simulink model "TP7_EJ3_espacio_estados"  (R2020a)
settings: Solver=VariableStepAuto  StartTime=0.0  StopTime=60  MaxStep=0.01  RelTol=1e-3
values from neighbouring files (symbols this model uses):
  A = [0 1 0 0 ... (first row only)    [TP7_EJ3_matrices.m]    (also in TP7_EJ6_matrices.m; TP7_EJ8.m)
  B = [0 0 0 1/m2]'    [TP7_EJ3_matrices.m]    (also in TP7_EJ6_matrices.m; TP7_EJ8.m = [0 0 0 k2/m2]')
  C1 = [1 0 0 0]    [TP7_EJ3_matrices.m]
  C2 = [0 0 1 0]    [TP7_EJ3_matrices.m]
  D = [0]    [TP7_EJ3_matrices.m]    (also in TP7_EJ6_matrices.m = [0;0]; TP7_EJ8.m = [0;0])
settings Model: Creator=LENOVO  LastModifiedBy=LENOVO

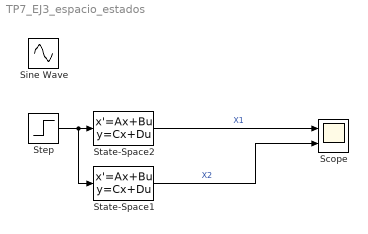
== system TP7_EJ3_espacio_estados ==
  Scope : Scope  NumInputPorts=2
  Sine Wave : Sin  SampleTime=0
  State-Space1 : StateSpace  A=A  B=B  C=C2  D=D  InitialCondition=0
  State-Space2 : StateSpace  A=A  B=B  C=C1  D=D  InitialCondition=0
  Step : Step  SampleTime=0
  wires:
  State-Space1/1 -> Scope/2  "X2"
  State-Space2/1 -> Scope/1  "X1"
  Step/1 -> State-Space1/1, State-Space2/1
